simulink model "part2_question1"  (R2023a)
settings: Solver=FixedStepDiscrete  StartTime=0.0  StopTime=150  RelTol=1e-3
settings Model: Creator=ma_kaba  LastModifiedBy=ma_kaba

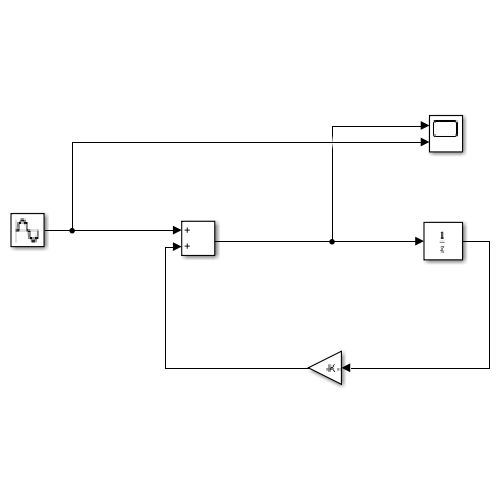
[thumbnail: Simulink's stored preview of the top-level diagram]
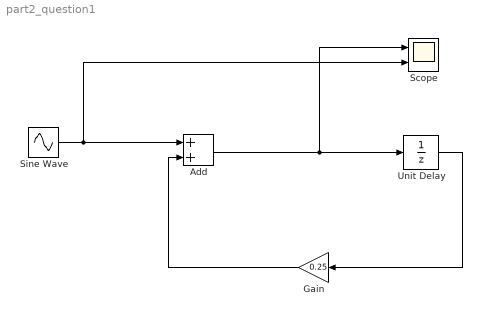
== system part2_question1 ==
  Add : Sum
  Gain : Gain  Gain=0.25
  Scope : Scope  NumInputPorts=2
  Sine Wave : Sin  Frequency=2*pi*(1/150)  SampleTime=5
  Unit Delay : UnitDelay  SampleTime=-1  HasFrameUpgradeWarning=on
  wires:
  Sine Wave/1 -> Scope/2, Add/1
  Add/1 -> Scope/1, Unit Delay/1
  Unit Delay/1 -> Gain/1
  Gain/1 -> Add/2
